simulink model "QuadRotorSystem_NoTune"  (R2014b)
settings: Solver=ode23t  StartTime=0.0  StopTime=15  RelTol=1e-3
undefined symbols (not defined in the file): Ap, getArbitraryAngle, getArbitraryAxis, kt, L, Pitch_0, rho, Roll_0, Rp, X, Y, Z, zInit
libraries: sm_lib x125, fl_lib x106, nesl_utility x49, elec_lib x12, simulink x6, aerolibtransform2 x4, aerolibconvert2 x2
(part 5 of 5)

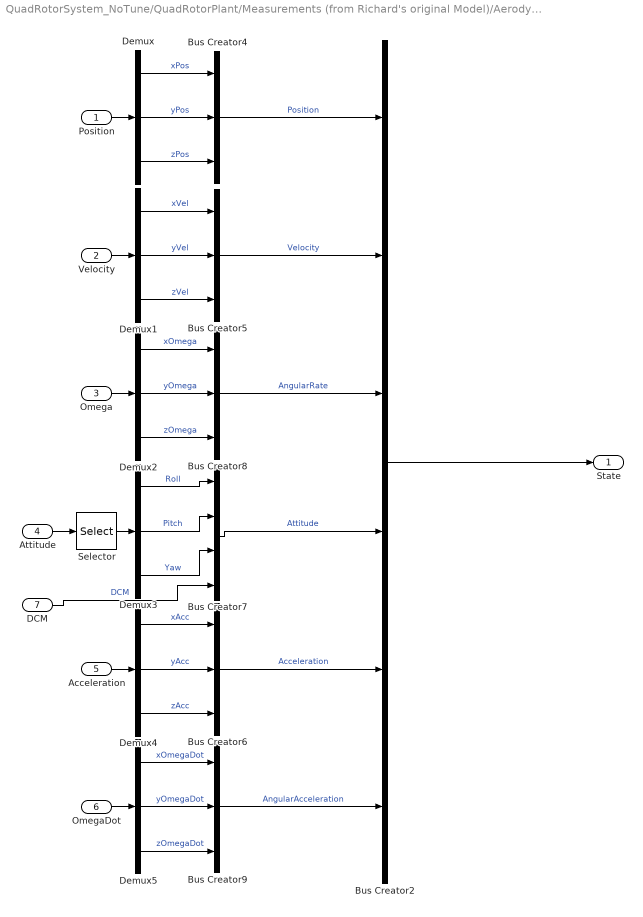
== system QuadRotorSystem_NoTune/QuadRotorPlant/Measurements (from Richard's original Model)/Aerodynamic Drag/World Data/Bus Mapping ==
  Position : Inport
  Velocity : Inport  Port=2
  Omega : Inport  Port=3
  Attitude : Inport  Port=4
  Acceleration : Inport  Port=5
  OmegaDot : Inport  Port=6
  DCM : Inport  Port=7
  Bus Creator2 : BusCreator  Inputs=6  OutDataTypeStr=Bus: States  NonVirtualBus=on
  Bus Creator4 : BusCreator  Inputs=3  OutDataTypeStr=Bus: PositionBus  NonVirtualBus=on
  Bus Creator5 : BusCreator  Inputs=3  OutDataTypeStr=Bus: VelocityBus  NonVirtualBus=on
  Bus Creator6 : BusCreator  Inputs=3  OutDataTypeStr=Bus: AccelerationBus  NonVirtualBus=on
  Bus Creator7 : BusCreator  OutDataTypeStr=Bus: AttitudeBus  NonVirtualBus=on
  Bus Creator8 : BusCreator  Inputs=3  OutDataTypeStr=Bus: AngularRateBus  NonVirtualBus=on
  Bus Creator9 : BusCreator  Inputs=3  OutDataTypeStr=Bus: AngularAccelerationBus  NonVirtualBus=on
  Demux{,1..5} (6 alike) : Demux  Outputs=3
  Selector : Selector  InputPortWidth=3  Indices=[3 2 1]
  State : Outport  OutDataTypeStr=Bus: States
  wires:
  DCM/1 -> Bus Creator7/4  "DCM"
  OmegaDot/1 -> Demux5/1
  Acceleration/1 -> Demux4/1
  Attitude/1 -> Selector/1
  Bus Creator2/1 -> State/1
  Omega/1 -> Demux2/1
  Velocity/1 -> Demux1/1
  Position/1 -> Demux/1
  Bus Creator9/1 -> Bus Creator2/6  "AngularAcceleration"
  Bus Creator6/1 -> Bus Creator2/5  "Acceleration"
  Bus Creator7/1 -> Bus Creator2/4  "Attitude"
  Bus Creator8/1 -> Bus Creator2/3  "AngularRate"
  Bus Creator5/1 -> Bus Creator2/2  "Velocity"
  Bus Creator4/1 -> Bus Creator2/1  "Position"
  Selector/1 -> Demux3/1
  Demux5/3 -> Bus Creator9/3  "zOmegaDot"
  Demux5/2 -> Bus Creator9/2  "yOmegaDot"
  Demux5/1 -> Bus Creator9/1  "xOmegaDot"
  Demux4/3 -> Bus Creator6/3  "zAcc"
  Demux4/2 -> Bus Creator6/2  "yAcc"
  Demux4/1 -> Bus Creator6/1  "xAcc"
  Demux2/3 -> Bus Creator8/3  "zOmega"
  Demux2/2 -> Bus Creator8/2  "yOmega"
  Demux2/1 -> Bus Creator8/1  "xOmega"
  Demux1/3 -> Bus Creator5/3  "zVel"
  Demux1/2 -> Bus Creator5/2  "yVel"
  Demux1/1 -> Bus Creator5/1  "xVel"
  Demux/3 -> Bus Creator4/3  "zPos"
  Demux/2 -> Bus Creator4/2  "yPos"
  Demux/1 -> Bus Creator4/1  "xPos"
  Demux3/1 -> Bus Creator7/1  "Roll"
  Demux3/3 -> Bus Creator7/3  "Yaw"
  Demux3/2 -> Bus Creator7/2  "Pitch"

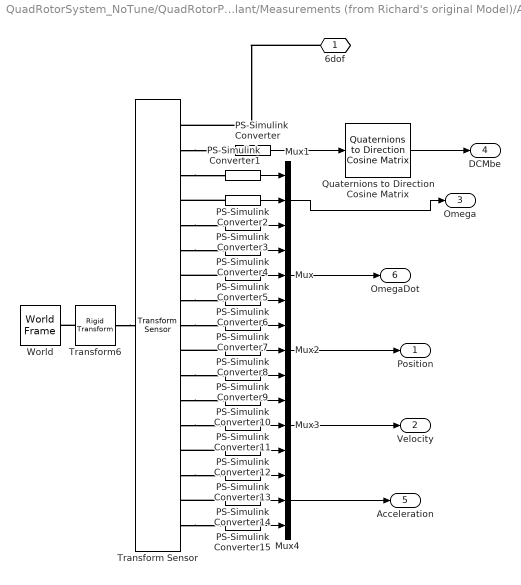
== system QuadRotorSystem_NoTune/QuadRotorPlant/Measurements (from Richard's original Model)/Aerodynamic Drag/World Data/Subsystem ==
  Mux{,1..4} (5 alike) : Mux  Inputs=3
  PS-Simulink Converter{,1..15} (16 alike) : nesl_utility/PS-Simulink Converter  PhysicalDomain=network_engine_domain  SubClassName=ps_output  LeftPortType=input  RightPortType=output  PseudoPeriodic=off  Frequencies=[]  Unit=1  AffineConversion=off
  Quaternions to Direction Cosine Matrix : aerolibtransform2/Quaternions to  Direction Cosine Matrix
  Transform Sensor : sm_lib/Frames and Transforms/Transform Sensor  MeasurementFrame=World  SenseAngle=off  SenseAxis=off  SenseAngle1=off  SenseAngle2=off  SenseAngle3=off  SenseQ=on  SenseR=off  SenseOmegaX=on  SenseOmegaY=on  SenseOmegaZ=on  SenseOmega1=off  SenseOmega2=off  SenseOmega3=off  SenseQDot=off  SenseRDot=off  SenseAlphaX=on  SenseAlphaY=on  SenseAlphaZ=on  SenseAlpha1=off  SenseAlpha2=off  SenseAlpha3=off  SenseQDDot=off  SenseRDDot=off  SenseX=on  SenseY=on  SenseZ=on  SenseRad=off  SenseAzim=off  SenseDist=off  SenseInc=off  SenseXDot=on  SenseYDot=on  SenseZDot=on  SenseRadDot=off  SenseAzimDot=off  SenseDistDot=off  SenseIncDot=off  SenseXDDot=on  SenseYDDot=on  SenseZDDot=on  SenseRadDDot=off  SenseAzimDDot=off  SenseDistDDot=off  SenseIncDDot=off  BlockFunction=simmechanics.library.frames_transforms.transform_sensor
  Transform6 : sm_lib/Frames and Transforms/Rigid Transform  TranslationMethod=None  TranslationLengthUnit=m  TranslationStandardAxis=+Z  TranslationStandardOffset=0  TranslationCartesianOffset=[0 0 0]  TranslationROffset=0  TranslationROffsetUnits=m  TranslationZOffset=0  TranslationZOffsetUnits=m  TranslationThetaOffset=0  TranslationThetaOffsetUnits=deg  RotationMethod=StandardAxis  RotationAngleUnits=deg  RotationStandardAxis=+X  RotationAngle=180  RotationArbitraryAxis=[0 0 1]  FollAlignAxisA=+X  BaseAlignAxisA=+Y  FollAlignAxisB=+Y  BaseAlignAxisB=+Z  RotationMatrix=[1 0 0; 0 1 0; 0 0 1]  BlockFunction=simmechanics.library.frames_transforms.rigid_transform
  World : sm_lib/Frames and Transforms/World Frame  BlockFunction=simmechanics.library.frames_transforms.world_frame
  "6dof " : PMIOPort  Port=1  Side=Left
  Position : Outport
  Velocity : Outport  Port=2
  Omega : Outport  Port=3
  DCMbe : Outport  Port=4
  Acceleration : Outport  Port=5
  OmegaDot : Outport  Port=6
  wires:
  PS-Simulink Converter5/1 -> Mux/2
  PS-Simulink Converter4/1 -> Mux/1
  PS-Simulink Converter9/1 -> Mux2/3
  PS-Simulink Converter7/1 -> Mux2/1
  PS-Simulink Converter6/1 -> Mux/3
  PS-Simulink Converter8/1 -> Mux2/2
  Quaternions to Direction Cosine Matrix/1 -> DCMbe/1
  PS-Simulink Converter14/1 -> Mux4/2
  PS-Simulink Converter15/1 -> Mux4/3
  PS-Simulink Converter13/1 -> Mux4/1
  PS-Simulink Converter12/1 -> Mux3/3
  PS-Simulink Converter11/1 -> Mux3/2
  PS-Simulink Converter10/1 -> Mux3/1
  PS-Simulink Converter3/1 -> Mux1/3
  PS-Simulink Converter2/1 -> Mux1/2
  PS-Simulink Converter1/1 -> Mux1/1
  PS-Simulink Converter/1 -> Quaternions to Direction Cosine Matrix/1
  Mux2/1 -> Position/1
  Mux3/1 -> Velocity/1
  Mux1/1 -> Omega/1
  Mux4/1 -> Acceleration/1
  Mux/1 -> OmegaDot/1
  connections:
  Transform6/RConn1 -- Transform Sensor/LConn1
  Transform6/LConn1 -- World/RConn1
  Transform Sensor/RConn17 -- PS-Simulink Converter15/LConn1
  Transform Sensor/RConn15 -- PS-Simulink Converter13/LConn1
  PS-Simulink Converter14/LConn1 -- Transform Sensor/RConn16
  Transform Sensor/RConn2 -- PS-Simulink Converter/LConn1
  PS-Simulink Converter2/LConn1 -- Transform Sensor/RConn4
  PS-Simulink Converter12/LConn1 -- Transform Sensor/RConn14
  Transform Sensor/RConn6 -- PS-Simulink Converter4/LConn1
  PS-Simulink Converter5/LConn1 -- Transform Sensor/RConn7
  Transform Sensor/RConn11 -- PS-Simulink Converter9/LConn1
  Transform Sensor/RConn13 -- PS-Simulink Converter11/LConn1
  "6dof "/RConn1 -- Transform Sensor/RConn1
  Transform Sensor/RConn5 -- PS-Simulink Converter3/LConn1
  Transform Sensor/RConn8 -- PS-Simulink Converter6/LConn1
  Transform Sensor/RConn3 -- PS-Simulink Converter1/LConn1
  PS-Simulink Converter8/LConn1 -- Transform Sensor/RConn10
  Transform Sensor/RConn12 -- PS-Simulink Converter10/LConn1
  Transform Sensor/RConn9 -- PS-Simulink Converter7/LConn1
